simulink model "sampleModel369"  (R2021b)
settings: Solver=VariableStepAuto  StartTime=0.0  StopTime=10.0  RelTol=1e-3
undefined symbols (not defined in the file or in its folder): DiscIntNeverNeededParam
libraries: simulink x8, slpidlib x1
settings Model: Creator=user  LastModifiedBy=user

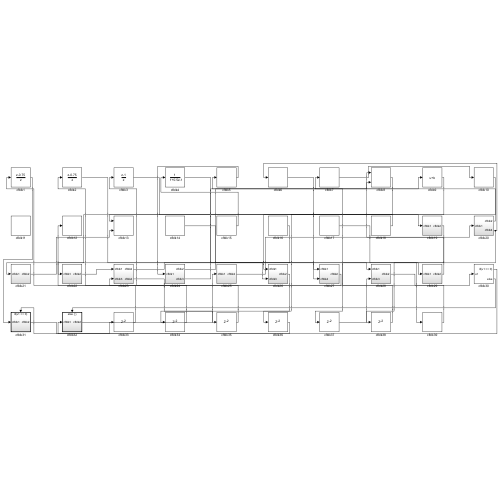
[thumbnail: Simulink's stored preview of the top-level diagram]
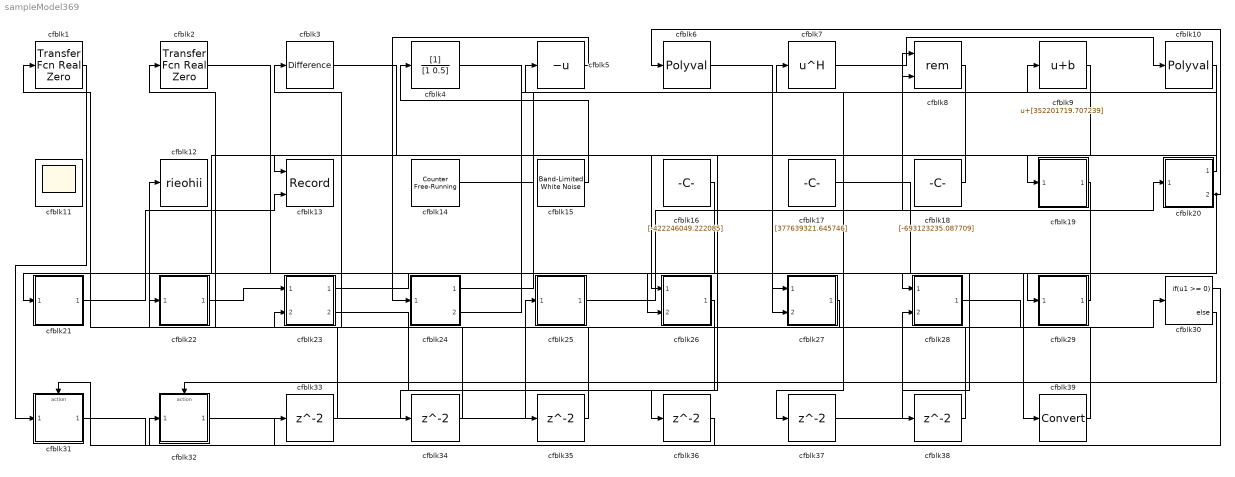
== system sampleModel369 ==
  cfblk1 : simulink/Discrete/Transfer Fcn Real Zero  ZeroZ=0.75  ICPrevInput=0.0  DoSatur=off
      settings: SourceProductBaseCode=SL
  cfblk10 : Polyval  Coefs=[ +2.081618890e-019, -1.441693666e-014, +4.719686976e-010, -8.536869453e-006, +1.621573104e-001, -8.087801117e+001 ]
  cfblk11 : Scope
      settings: Floating=on
  cfblk12 : ToWorkspace  VariableName=rieohii  SaveFormat=Timeseries  SampleTime=-1
  cfblk13 : Record  FileSettingsInternal="{\"entries\":[{\"content\":{\"excelSettings\":{\"content\":{},\"type\":\"Streamout.ExcelSettings\"}},\"type\":\"Streamout.FileSettingStorage\",\"uuid\":\"5e07db8c-c53c-4203-a8f2-b89d4bef93c7\"}],\"packageUris\":[\"http://schema.mathworks.com/mf0/streamout_blocks/R2020a\"],\"version\":\"1.0\"}"  Layout=[1 1]  SignalsInternal="{\"entries\":[{\"content\":{\"signals\":[{\"content\":{\"blockPath\":[\"sampleModel369/cfblk13\"],\"channel\":[],\"dimensions\":[1],\"domain\":\"sampleModel369/cfblk13\",\"lineColor\":\"#a2142f\",\"plots\":[1],\"port\":1,\"sid\":[\"\"],\"signalID\":15293,\"signalName\":\"cfblk18\"},\"type\":\"RecordBlkView.Signal\",\"uuid\":\"efcfa3d0-b0d7-471d-84cf-30bcc8451d86\"},{\"content\":{\"blockPath\":[\"sampleModel369/cfblk13\"],\"channel\":[],\"dimensions\":[1],\"domain\":\"sampleModel369/cfblk13\",\"lineColor\":\"#139fff\",\"plots\":[1],\"port\":2,\"sid\":[\"\"],\"signalID\":15297,\"signalName\":\"cfblk21\"},\"type\":\"RecordBlkView.Signal\",\"uuid\":\"47b736da-b121-4262-af2f-0a21b28e4ce5\"}]},\"type\":\"RecordBlkView.InputSignals\",\"uuid\":\"d274cc77-b9e7-4892-9679-ea18a9c4d1c2\"}],\"packageUris\":[\"http://schema.mathworks.com/mf0/streamout_blocks/R2020a\"],\"version\":\"1.0\"}"  VisualizationBindings="{\"xyplotplugin\":{\"info\":[{\"series\":[{\"bindingParametersList\":[{\"parameter\":\"X-Axis\",\"signalID\":15293,\"signalName\":\"cfblk18\"},{\"parameter\":\"Y-Axis\",\"signalID\":15297,\"signalName\":\"cfblk21\"}],\"seriesID\":28960}],\"subplotID\":1}]}}"  CompatibilityTag=XY
  cfblk14 : simulink/Sources/Counter Free-Running  NumBits=[45.000000]  tsamp=-1
  cfblk15 : simulink/Sources/Band-Limited White Noise  Cov=[7705343364.445023]  Ts=0.1  seed=[7549194394.000000]
  cfblk16 : Constant  Value=[-422246049.222085]  SampleTime=1
  cfblk17 : Constant  Value=[377639321.645746]  SampleTime=1
  cfblk18 : Constant  Value=[-693123235.087709]  SampleTime=1
  cfblk19 : Subsystem
  cfblk2 : simulink/Discrete/Transfer Fcn Real Zero  ZeroZ=0.75  ICPrevInput=0.0  DoSatur=off
      settings: SourceProductBaseCode=SL
  cfblk20 : Subsystem
  cfblk21 : Subsystem
  cfblk22 : Subsystem
  cfblk23 : Subsystem
  cfblk24 : Subsystem
  cfblk25 : Subsystem
  cfblk26 : Subsystem
  cfblk27 : Subsystem
  cfblk28 : Subsystem
  cfblk29 : Subsystem
  cfblk3 : simulink/Discrete/Difference  ICPrevInput=0.0  OutMin=[]  OutMax=[]  OutDataTypeStr=Inherit: Inherit via back propagation  OutDataType=fixdt(1, 16)  OutScaling=2^-10  DoSatur=off
  cfblk30 : If  IfExpression=u1 >= 0  SampleTime=1
  cfblk31 : Subsystem  TreatAsAtomicUnit=on
  cfblk32 : Subsystem  TreatAsAtomicUnit=on
  cfblk{33..38} (6 alike) : Delay  SampleTime=1
  cfblk39 : DataTypeConversion
  cfblk4 : DiscreteFilter  SampleTime=1
  cfblk5 : UnaryMinus
  cfblk6 : Polyval  Coefs=[ +2.081618890e-019, -1.441693666e-014, +4.719686976e-010, -8.536869453e-006, +1.621573104e-001, -8.087801117e+001 ]
  cfblk7 : Math  Operator=hermitian  SaturateOnIntegerOverflow=on
  cfblk8 : Math  Operator=rem  SaturateOnIntegerOverflow=on
  cfblk9 : Bias  Bias=[352201719.707239]
  wires:
  cfblk20/1(cfblk2) -> cfblk5/1
  cfblk25/1(cfblk2) -> cfblk20/1(cfblk1)
  cfblk17/1 -> cfblk29/1(cfblk1)
  cfblk28/1(cfblk2) -> cfblk30/1
  cfblk15/1 -> cfblk4/1
  cfblk5/1 -> cfblk24/1(cfblk1)
  cfblk27/1(cfblk2) -> cfblk12/1
  cfblk32/1(cfblk2) -> cfblk25/1(cfblk1)
  cfblk16/1 -> cfblk21/1(cfblk1)
  cfblk7/1 -> cfblk10/1
  cfblk1/1 -> cfblk31/1(cfblk1)
  cfblk22/1(cfblk2) -> cfblk23/1(cfblk1)
  cfblk8/1 -> cfblk22/1(cfblk1)
  cfblk29/1(cfblk2) -> cfblk8/1
  cfblk24/1(cfblk2) -> cfblk8/2
  cfblk6/1 -> cfblk27/1(cfblk1)
  cfblk10/1 -> cfblk26/1(cfblk1)
  cfblk3/1 -> cfblk19/1(cfblk1)
  cfblk18/1 -> cfblk13/1
  cfblk24/2(cfblk3) -> cfblk9/1
  cfblk21/1(cfblk2) -> cfblk13/2
  cfblk2/1 -> cfblk28/1(cfblk1)
  cfblk20/2(cfblk4) -> cfblk6/1, cfblk37/1
  cfblk23/1(cfblk2) -> cfblk26/2(cfblk3)
  cfblk4/1 -> cfblk27/2(cfblk4)
  cfblk30/1 -> cfblk31/Action
  cfblk30/2 -> cfblk32/Action
  cfblk31/1(cfblk2) -> cfblk33/1
  cfblk33/1 -> cfblk1/1
  cfblk26/1(cfblk2) -> cfblk34/1
  cfblk34/1 -> cfblk23/2(cfblk3)
  cfblk23/2(cfblk4) -> cfblk35/1
  cfblk35/1 -> cfblk2/1
  cfblk9/1 -> cfblk36/1
  cfblk36/1 -> cfblk32/1(cfblk1)
  cfblk37/1 -> cfblk28/2(cfblk3)
  cfblk19/1(cfblk2) -> cfblk38/1
  cfblk38/1 -> cfblk3/1
  cfblk14/1 -> cfblk39/1
  cfblk39/1 -> cfblk7/1

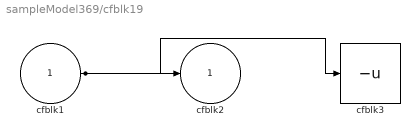
== system sampleModel369/cfblk19 ==
  cfblk1 : Inport
  cfblk3 : UnaryMinus
  cfblk2 : Outport
  wires:
  cfblk1/1 -> cfblk2/1, cfblk3/1

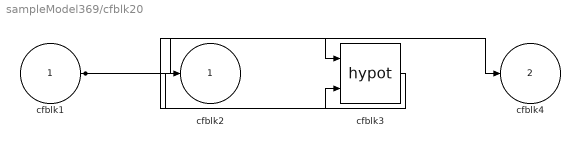
== system sampleModel369/cfblk20 ==
  cfblk1 : Inport
  cfblk3 : Math  Operator=hypot  SaturateOnIntegerOverflow=on
  cfblk2 : Outport
  cfblk4 : Outport  Port=2
  wires:
  cfblk1/1 -> cfblk4/1, cfblk3/1, cfblk3/2
  cfblk3/1 -> cfblk2/1

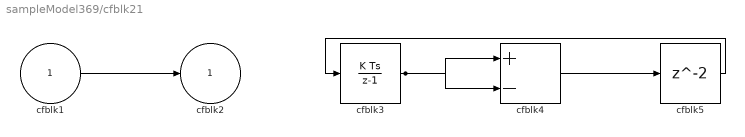
== system sampleModel369/cfblk21 ==
  cfblk1 : Inport
  cfblk3 : DiscreteIntegrator  ICPrevOutput=DiscIntNeverNeededParam  ICPrevScaledInput=DiscIntNeverNeededParam
  cfblk4 : Sum  Inputs=+-
  cfblk5 : Delay  SampleTime=1
  cfblk2 : Outport
  wires:
  cfblk1/1 -> cfblk2/1
  cfblk3/1 -> cfblk4/1, cfblk4/2
  cfblk4/1 -> cfblk5/1
  cfblk5/1 -> cfblk3/1

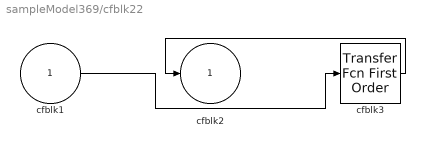
== system sampleModel369/cfblk22 ==
  cfblk1 : Inport
  cfblk3 : simulink/Discrete/Transfer Fcn First Order  PoleZ=0.95  ICPrevOutput=0.0  DoSatur=off
  cfblk2 : Outport
  wires:
  cfblk3/1 -> cfblk2/1
  cfblk1/1 -> cfblk3/1

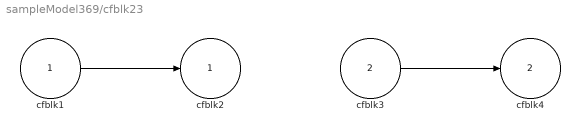
== system sampleModel369/cfblk23 ==
  cfblk1 : Inport
  cfblk3 : Inport  Port=2
  cfblk2 : Outport
  cfblk4 : Outport  Port=2
  wires:
  cfblk3/1 -> cfblk4/1
  cfblk1/1 -> cfblk2/1

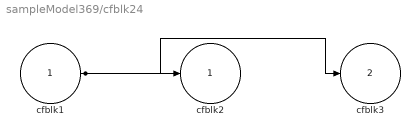
== system sampleModel369/cfblk24 ==
  cfblk1 : Inport
  cfblk2 : Outport
  cfblk3 : Outport  Port=2
  wires:
  cfblk1/1 -> cfblk2/1, cfblk3/1

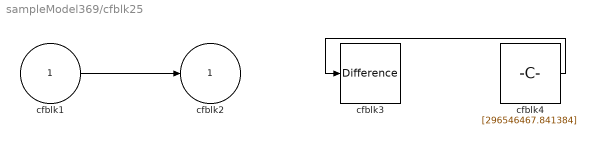
== system sampleModel369/cfblk25 ==
  cfblk1 : Inport
  cfblk3 : simulink/Discrete/Difference  ICPrevInput=0.0  OutMin=[]  OutMax=[]  OutDataTypeStr=Inherit: Inherit via back propagation  OutDataType=fixdt(1, 16)  OutScaling=2^-10  DoSatur=off
  cfblk4 : Constant  Value=[296546467.841384]  SampleTime=1
  cfblk2 : Outport
  wires:
  cfblk1/1 -> cfblk2/1
  cfblk4/1 -> cfblk3/1

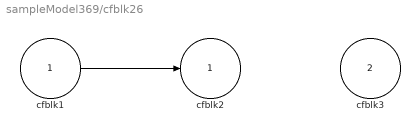
== system sampleModel369/cfblk26 ==
  cfblk1 : Inport
  cfblk3 : Inport  Port=2
  cfblk2 : Outport
  wires:
  cfblk1/1 -> cfblk2/1

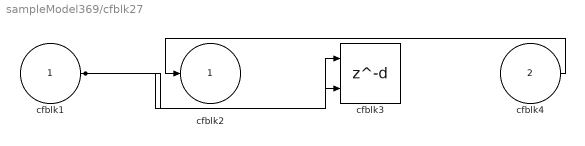
== system sampleModel369/cfblk27 ==
  cfblk1 : Inport
  cfblk4 : Inport  Port=2
  cfblk3 : Delay  DelayLengthSource=Input port  SampleTime=1
      settings: InputPortMap=u0,p1
  cfblk2 : Outport
  wires:
  cfblk4/1 -> cfblk2/1
  cfblk1/1 -> cfblk3/1, cfblk3/2

== system sampleModel369/cfblk28 ==
  cfblk1 : Inport
  cfblk3 : Inport  Port=2
  cfblk2 : Outport
  wires:
  cfblk3/1 -> cfblk2/1

== system sampleModel369/cfblk29 ==
  cfblk1 : Inport
  cfblk3 : Constant  Value=[574963328.278269]  SampleTime=1
  cfblk2 : Outport
  wires:
  cfblk1/1 -> cfblk2/1

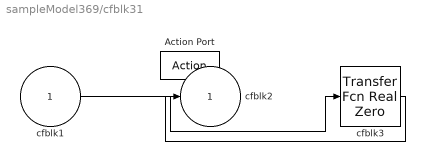
== system sampleModel369/cfblk31 ==
  cfblk1 : Inport
  Action Port : ActionPort  ActionPortLabel=if(u1 >= 0)
  cfblk3 : simulink/Discrete/Transfer Fcn Real Zero  ZeroZ=0.75  ICPrevInput=0.0  DoSatur=off
      settings: SourceProductBaseCode=SL
  cfblk2 : Outport
  wires:
  cfblk1/1 -> cfblk3/1
  cfblk3/1 -> cfblk2/1

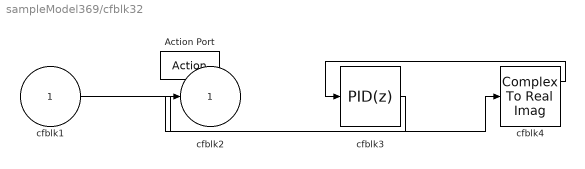
== system sampleModel369/cfblk32 ==
  cfblk1 : Inport
  Action Port : ActionPort  ActionPortLabel=else
  cfblk3 : slpidlib/PID Controller  Controller=PID  Form=Parallel  TimeDomain=Discrete-time  UseExternalTs=off  SampleTime=-1  IntegratorMethod=Forward Euler  FilterMethod=Forward Euler  ControllerParametersSource=internal  P=1  I=1  D=0  UseFilter=on  N=100  TunerSelectOption=Transfer Function Based (PID Tuner App)  InitialConditionSource=internal  InitialConditionForIntegrator=0  InitialConditionForFilter=0  DifferentiatorICPrevScaledInput=0  ExternalReset=none  TrackingMode=off  Kt=1  LimitOutput=off  SatLimitsSource=internal  UpperSaturationLimit=inf  LowerSaturationLimit=-inf  LinearizeAsGain=off  AntiWindupMode=none  Kb=1  POutMin=[]  POutMax=[]  IOutMin=[]  IOutMax=[]  DOutMin=[]  DOutMax=[]  NOutMin=[]  NOutMax=[]  SumOutMin=[]  SumOutMax=[]  SaturationOutMin=[]  SaturationOutMax=[]  PParamMin=[]  PParamMax=[]  IParamMin=[]  IParamMax=[]  DParamMin=[]  DParamMax=[]  NParamMin=[]  NParamMax=[]  KbParamMin=[]  KbParamMax=[]  KtParamMin=[]  KtParamMax=[]  KbOutMin=[]  KbOutMax=[]  KtOutMin=[]  KtOutMax=[]  IntegratorOutMin=[]  IntegratorOutMax=[]  FilterOutMin=[]  FilterOutMax=[]  SumI1OutMin=[]  SumI1OutMax=[]  SumI2OutMin=[]  SumI2OutMax=[]  SumI3OutMin=[]  SumI3OutMax=[]  SumI4OutMin=[]  SumI4OutMax=[]  SumDOutMin=[]  SumDOutMax=[]  DifferentiatorOutMin=[]  DifferentiatorOutMax=[]  FilterDiffOutCoefMin=[]  FilterDiffOutCoefMax=[]  ReciprocalOutMin=[]  ReciprocalOutMax=[]  SumDenOutMin=[]  SumDenOutMax=[]  SumNumOutMin=[]  SumNumOutMax=[]  DivideOutMin=[]  DivideOutMax=[]  UdiffTsProdOutMin=[]  UdiffTsProdOutMax=[]  NTsProdOutMin=[]  NTsProdOutMax=[]  UintegralTsProdOutMin=[]  UintegralTsProdOutMax=[]  UngainTsProdOutMin=[]  UngainTsProdOutMax=[]  IntegratorContinuousStateAttributes=''  IntegratorStateMustResolveToSignalObject=off  IntegratorRTWStateStorageClass=Auto  FilterContinuousStateAttributes=''  FilterStateMustResolveToSignalObject=off  FilterRTWStateStorageClass=Auto  ParallelPVariant=InternalParameters  IdealPVariant=Disabled  IVariant=InternalParameters  DVariant=InternalParameters  IntegratorVariant=Discrete  SatVariant=Disabled  AWVariant=Passthrough  PCopyVariant=Disabled  TRVariant=Disabled  FdbkBlocksVariant=Forward  IdealPFdbkVariant=Disabled  SatFdbkVariant=Disabled  DerivativeFilterVariant=ForwardEulerFilter  NVariant=InternalParameters  NCopyVariant=Disabled  FilterICVariant=InternalICsFilter  IntegratorICVariant=InternalICs  ExternalResetVariant=Disabled  TRSumVariant=Passthrough  SumFdbkVariant=Disabled  SumVariant=Sum_PID  TsampFilterVariant=InternalTs  TsampNgainVariant=Passthrough  TsampIntegralVariant=Passthrough  ExternalSaturationOutDataTypeStr=Inherit: Same as second input
  cfblk4 : ComplexToRealImag
  cfblk2 : Outport
  wires:
  cfblk1/1 -> cfblk4/1
  cfblk4/1 -> cfblk3/1
  cfblk3/1 -> cfblk2/1
